simulink model "ebike_UB_2"  (Simulink 8.5)
settings: Solver=ode3  StartTime=0.0  StopTime=0.5  FixedStep=0.001  MaxStep=0.001  MinStep=0.001  RelTol=1e-3
values from neighbouring files (symbols this model uses):
  air_density = 1.225    [run_sim.m]
  air_drag_coeff = 0.4    [run_sim.m]
  frontal_area = 0.38    [run_sim.m]
  gravity = 9.8    [run_sim.m]
  rolling_fric_coeff = 0.003    [run_sim.m]
  vehicle_mass = driver_mass+bike_mass    (= 82)    [run_sim.m]
libraries: simulink x1
settings Model: Creator=stwei  LastModifiedBy=bolatu
settings DataIOCC: SignalLoggingSaveFormat=Dataset  SaveOutput=off  ReturnWorkspaceOutputs=on
settings DebuggingCC: SolverPrmCheckMsg=warning  FcnCallInpInsideContextMsg=UseLocalSettings

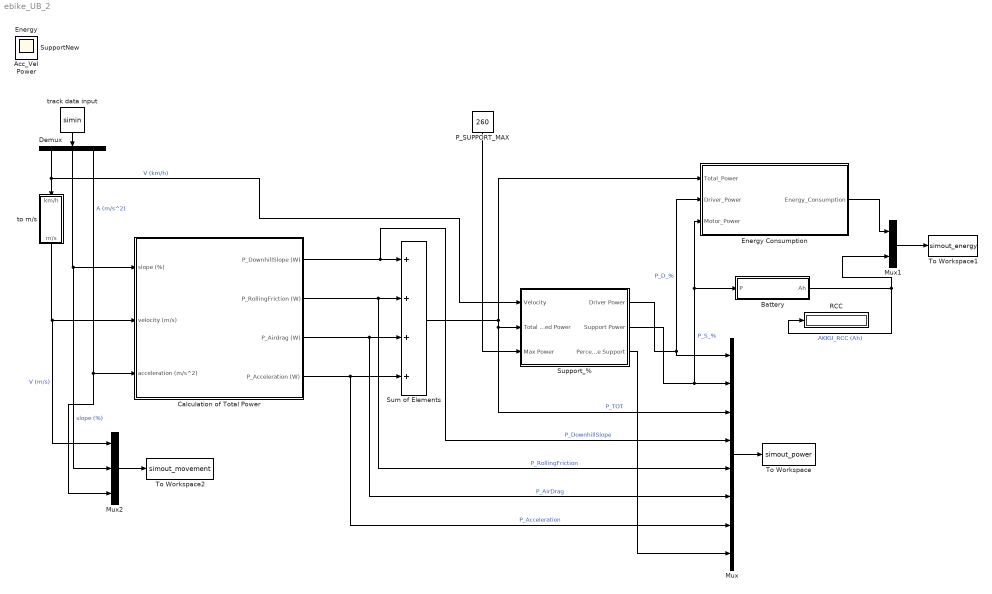
== system ebike_UB_2 ==
  Battery : Subsystem
  Calculation of Total Power : Subsystem
  Demux : Demux  Outputs=3
  Energy Consumption : Subsystem
  Mux : Mux  Inputs=8
  Mux1 : Mux  Inputs=2
  Mux2 : Mux  Inputs=3
  P_SUPPORT_MAX : Constant  Value=260
  RCC : Display
  Sum of Elements : Sum  Inputs=++++
  Support_% : Subsystem
  To Workspace : ToWorkspace  VariableName=simout_power  SaveFormat=Timeseries  SampleTime=-1
  To Workspace1 : ToWorkspace  VariableName=simout_energy  SaveFormat=Timeseries  SampleTime=-1
  To Workspace2 : ToWorkspace  VariableName=simout_movement  SaveFormat=Timeseries  SampleTime=-1
  to m/s : Subsystem
  track data input : FromWorkspace  VariableName=simin  SampleTime=0  OutputAfterFinalValue=Setting to zero
  Acc_Vel : Scope  NumInputPorts=4
      settings: ShowLegends=on  YMin=-5~-5~-5~-5  YMax=5~5~5~5
  Energy : Scope
      settings: ShowLegends=on  SaveName=ScopeData2
  Power : Scope
      settings: ShowLegends=on
  SupportNew : Scope  NumInputPorts=3
      settings: ShowLegends=on  YMin=-5~-5~-5  YMax=5~5~5  SaveName=ScopeData3
  wires:
  P_SUPPORT_MAX/1 -> Support_%/3(Max Power)
  track data input/1 -> Demux/1
  Demux/1 -> to m/s/1(km/h), Support_%/1(Velocity)  "V (km/h)"
  Demux/2 -> Mux2/2, Calculation of Total Power/1(slope (%))  "slope (%)"
  to m/s/1(m/s) -> Mux2/1, Calculation of Total Power/2(velocity (m/s))  "V (m/s)"
  Sum of Elements/1 -> Mux/3, Support_%/2(Total Needed Power), Energy Consumption/1(Total_Power)  "P_TOT"
  Calculation of Total Power/1(P_DownhillSlope (W)) -> Mux/4, Sum of Elements/1  "P_DownhillSlope"
  Calculation of Total Power/2(P_RollingFriction (W)) -> Mux/5, Sum of Elements/2  "P_RollingFriction"
  Calculation of Total Power/3(P_Airdrag (W)) -> Mux/6, Sum of Elements/3  "P_AirDrag"
  Calculation of Total Power/4(P_Acceleration (W)) -> Mux/7, Sum of Elements/4  "P_Acceleration"
  Demux/3 -> Mux2/3, Calculation of Total Power/3(acceleration (m/s^2))  "A (m/s^2)"
  Mux/1 -> To Workspace/1
  Support_%/2(Support Power) -> Energy Consumption/3(Motor_Power), Battery/1(P), Mux/2  "P_S_%"
  Support_%/1(Driver Power) -> Mux/1, Energy Consumption/2(Driver_Power)  "P_D_%"
  Energy Consumption/1(Energy_Consumption) -> Mux1/1
  Battery/1(Ah) -> RCC/1, Mux1/2  "AKKU_RCC (Ah)"
  Mux1/1 -> To Workspace1/1
  Mux2/1 -> To Workspace2/1
  Support_%/3(Percentage Support) -> Mux/8

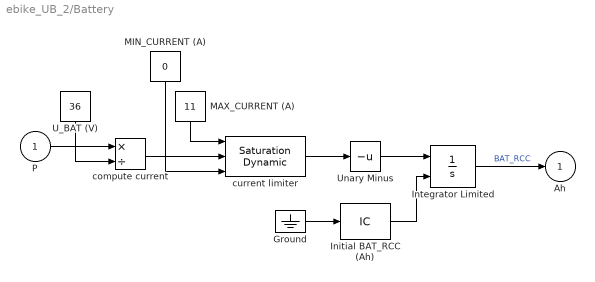
== system ebike_UB_2/Battery ==
  P : Inport
  Ground : Ground
  Initial BAT_RCC (Ah) : InitialCondition  Value=11
  Integrator Limited : Integrator  InitialConditionSource=external  LimitOutput=on  UpperSaturationLimit=13  LowerSaturationLimit=0
  MAX_CURRENT (A) : Constant  Value=11
  MIN_CURRENT (A) : Constant  Value=0
  U_BAT (V) : Constant  Value=36
  Unary Minus : UnaryMinus
  compute current : Product  Inputs=*/
  current limiter : simulink/Discontinuities/Saturation Dynamic  OutMin=[]  OutMax=[]  OutDataTypeStr=Inherit: Same as second input  OutDataType=fixdt(1, 16)  OutScaling=2^-10  DoSatur=on
  Ah : Outport
  wires:
  Ground/1 -> Initial BAT_RCC (Ah)/1
  U_BAT (V)/1 -> compute current/2
  Initial BAT_RCC (Ah)/1 -> Integrator Limited/2
  Unary Minus/1 -> Integrator Limited/1
  P/1 -> compute current/1
  Integrator Limited/1 -> Ah/1  "BAT_RCC"
  current limiter/1 -> Unary Minus/1
  compute current/1 -> current limiter/2
  MAX_CURRENT (A)/1 -> current limiter/1
  MIN_CURRENT (A)/1 -> current limiter/3

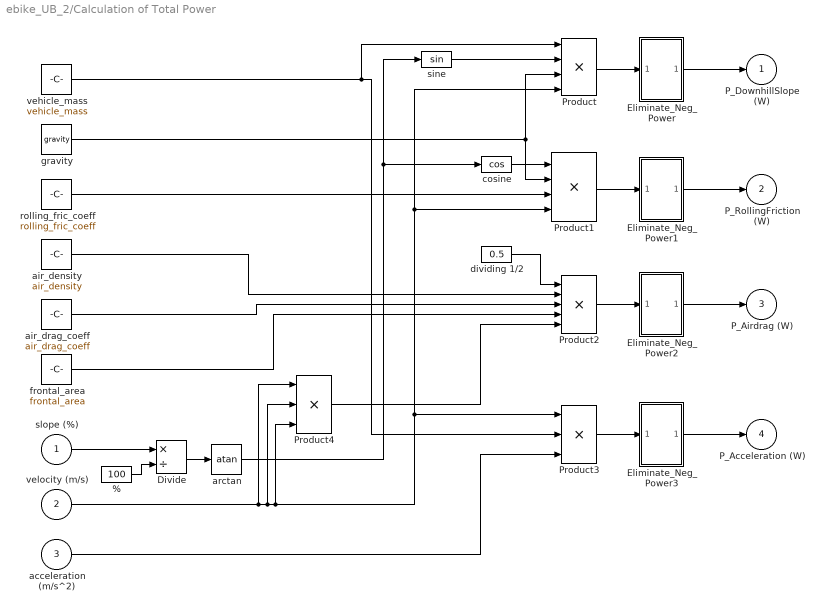
== system ebike_UB_2/Calculation of Total Power ==
  slope (%) : Inport
  velocity (m/s) : Inport  Port=2
  acceleration (m/s^2) : Inport  Port=3
  % : Constant  Value=100
  Divide : Product  Inputs=*/
  Eliminate_Neg_Power : Subsystem
  Eliminate_Neg_Power1 : Subsystem
  Eliminate_Neg_Power2 : Subsystem
  Eliminate_Neg_Power3 : Subsystem
  Product : Product  Inputs=4
  Product1 : Product  Inputs=4
  Product2 : Product  Inputs=5
  Product3 : Product  Inputs=3
  Product4 : Product  Inputs=3
  air_density : Constant  Value=air_density
  air_drag_coeff : Constant  Value=air_drag_coeff
  arctan : Trigonometry  Operator=atan
  cosine : Trigonometry  Operator=cos
  dividing 1/2 : Constant  Value=0.5
  frontal_area : Constant  Value=frontal_area
  gravity : Constant  Value=gravity
  rolling_fric_coeff : Constant  Value=rolling_fric_coeff
  sine : Trigonometry
  vehicle_mass : Constant  Value=vehicle_mass
  P_DownhillSlope (W) : Outport
  P_RollingFriction (W) : Outport  Port=2
  P_Airdrag (W) : Outport  Port=3
  P_Acceleration (W) : Outport  Port=4
  wires:
  slope (%)/1 -> Divide/1
  %/1 -> Divide/2
  Divide/1 -> arctan/1
  vehicle_mass/1 -> Product/1, Product3/2
  gravity/1 -> Product/3, Product1/2
  sine/1 -> Product/2
  arctan/1 -> sine/1, cosine/1
  velocity (m/s)/1 -> Product3/1, Product/4, Product1/4, Product4/3, Product4/2, Product4/1
  Product1/1 -> Eliminate_Neg_Power1/1(In1)
  cosine/1 -> Product1/1
  rolling_fric_coeff/1 -> Product1/3
  acceleration (m/s^2)/1 -> Product3/3
  air_density/1 -> Product2/2
  air_drag_coeff/1 -> Product2/3
  frontal_area/1 -> Product2/4
  Product4/1 -> Product2/5
  dividing 1/2/1 -> Product2/1
  Product/1 -> Eliminate_Neg_Power/1(In1)
  Eliminate_Neg_Power/1(Out1) -> P_DownhillSlope (W)/1
  Eliminate_Neg_Power1/1(Out1) -> P_RollingFriction (W)/1
  Product2/1 -> Eliminate_Neg_Power2/1(In1)
  Eliminate_Neg_Power2/1(Out1) -> P_Airdrag (W)/1
  Product3/1 -> Eliminate_Neg_Power3/1(In1)
  Eliminate_Neg_Power3/1(Out1) -> P_Acceleration (W)/1

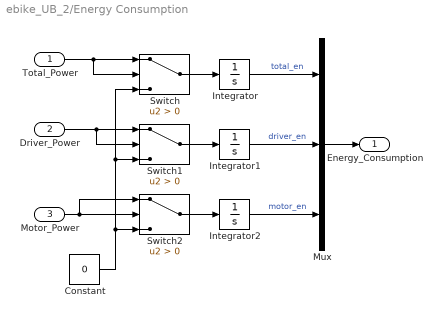
== system ebike_UB_2/Energy Consumption ==
  Total_Power : Inport
  Driver_Power : Inport  Port=2
  Motor_Power : Inport  Port=3
  Constant : Constant  Value=0
  Integrator : Integrator
  Integrator1 : Integrator
  Integrator2 : Integrator
  Mux : Mux  Inputs=3
  Switch : Switch  Criteria=u2 > Threshold
  Switch1 : Switch  Criteria=u2 > Threshold
  Switch2 : Switch  Criteria=u2 > Threshold
  Energy_Consumption : Outport
  wires:
  Switch2/1 -> Integrator2/1
  Switch1/1 -> Integrator1/1
  Switch/1 -> Integrator/1
  Integrator/1 -> Mux/1  "total_en"
  Integrator1/1 -> Mux/2  "driver_en"
  Integrator2/1 -> Mux/3  "motor_en"
  Mux/1 -> Energy_Consumption/1
  Total_Power/1 -> Switch/2, Switch/1
  Driver_Power/1 -> Switch1/2, Switch1/1
  Motor_Power/1 -> Switch2/1, Switch2/2
  Constant/1 -> Switch/3, Switch1/3, Switch2/3

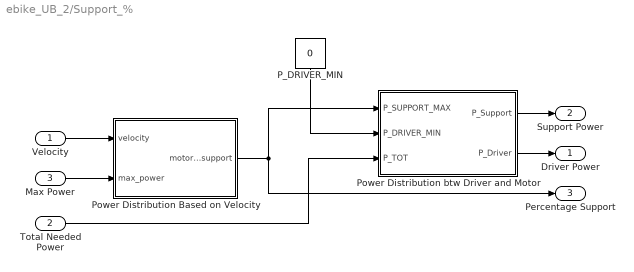
== system ebike_UB_2/Support_% ==
  Velocity : Inport
  Total Needed Power : Inport  Port=2
  Max Power : Inport  Port=3
  P_DRIVER_MIN : Constant  Value=0
  Power Distribution Based on Velocity : Subsystem
  Power Distribution btw Driver and Motor : Subsystem
  Driver Power : Outport
  Support Power : Outport  Port=2
  Percentage Support : Outport  Port=3
  wires:
  Total Needed Power/1 -> Power Distribution btw Driver and Motor/3(P_TOT)
  P_DRIVER_MIN/1 -> Power Distribution btw Driver and Motor/2(P_DRIVER_MIN)
  Power Distribution Based on Velocity/1(motor_support) -> Power Distribution btw Driver and Motor/1(P_SUPPORT_MAX), Percentage Support/1
  Power Distribution btw Driver and Motor/1(P_Support) -> Support Power/1
  Power Distribution btw Driver and Motor/2(P_Driver) -> Driver Power/1
  Max Power/1 -> Power Distribution Based on Velocity/2(max_power)
  Velocity/1 -> Power Distribution Based on Velocity/1(velocity)

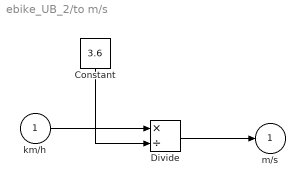
== system ebike_UB_2/to m/s ==
  km/h : Inport
  Constant : Constant  Value=3.6
  Divide : Product  Inputs=*/
  m/s : Outport
  wires:
  Constant/1 -> Divide/2
  km/h/1 -> Divide/1
  Divide/1 -> m/s/1

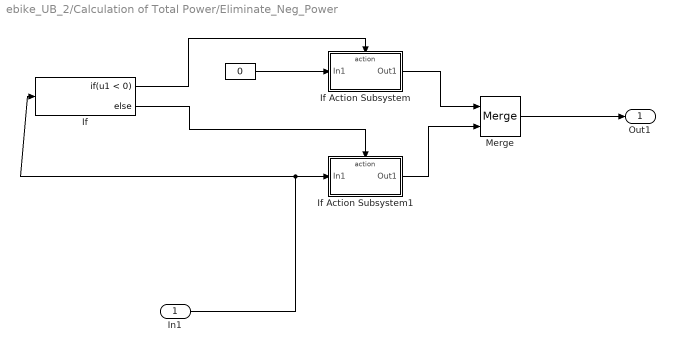
== system ebike_UB_2/Calculation of Total Power/Eliminate_Neg_Power ==
  In1 : Inport
  " " : Constant  Value=0
  If : If  IfExpression=u1 < 0
  If Action Subsystem : Subsystem  TreatAsAtomicUnit=on
  If Action Subsystem1 : Subsystem  TreatAsAtomicUnit=on
  Merge : Merge
  Out1 : Outport
  wires:
  If Action Subsystem1/1(Out1) -> Merge/2
  If/2 -> If Action Subsystem1/Action
  If Action Subsystem/1(Out1) -> Merge/1
  Merge/1 -> Out1/1
  " "/1 -> If Action Subsystem/1(In1)
  In1/1 -> If Action Subsystem1/1(In1), If/1
  If/1 -> If Action Subsystem/Action

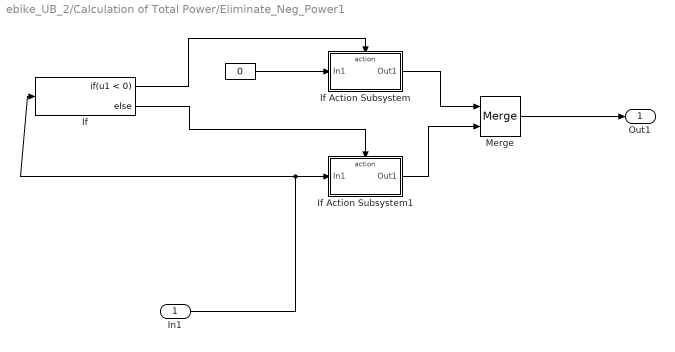
== system ebike_UB_2/Calculation of Total Power/Eliminate_Neg_Power1 ==
  In1 : Inport
  " " : Constant  Value=0
  If : If  IfExpression=u1 < 0
  If Action Subsystem : Subsystem  TreatAsAtomicUnit=on
  If Action Subsystem1 : Subsystem  TreatAsAtomicUnit=on
  Merge : Merge
  Out1 : Outport
  wires:
  If Action Subsystem1/1(Out1) -> Merge/2
  If/2 -> If Action Subsystem1/Action
  If Action Subsystem/1(Out1) -> Merge/1
  Merge/1 -> Out1/1
  " "/1 -> If Action Subsystem/1(In1)
  In1/1 -> If Action Subsystem1/1(In1), If/1
  If/1 -> If Action Subsystem/Action

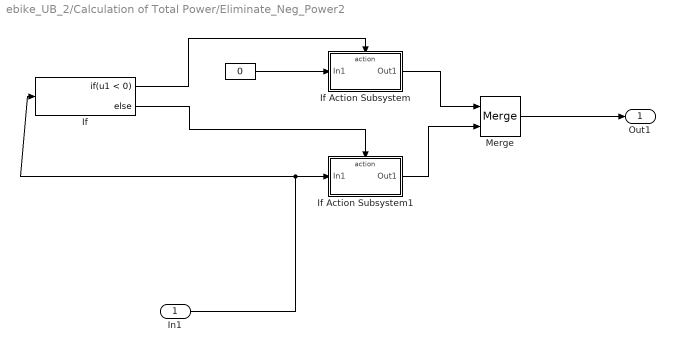
== system ebike_UB_2/Calculation of Total Power/Eliminate_Neg_Power2 ==
  In1 : Inport
  " " : Constant  Value=0
  If : If  IfExpression=u1 < 0
  If Action Subsystem : Subsystem  TreatAsAtomicUnit=on
  If Action Subsystem1 : Subsystem  TreatAsAtomicUnit=on
  Merge : Merge
  Out1 : Outport
  wires:
  If Action Subsystem1/1(Out1) -> Merge/2
  If/2 -> If Action Subsystem1/Action
  If Action Subsystem/1(Out1) -> Merge/1
  Merge/1 -> Out1/1
  " "/1 -> If Action Subsystem/1(In1)
  In1/1 -> If Action Subsystem1/1(In1), If/1
  If/1 -> If Action Subsystem/Action

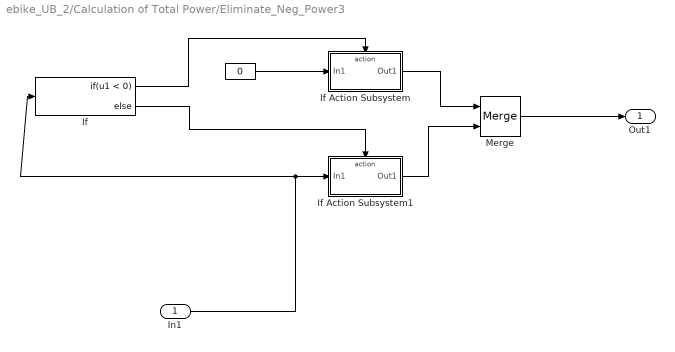
== system ebike_UB_2/Calculation of Total Power/Eliminate_Neg_Power3 ==
  In1 : Inport
  " " : Constant  Value=0
  If : If  IfExpression=u1 < 0
  If Action Subsystem : Subsystem  TreatAsAtomicUnit=on
  If Action Subsystem1 : Subsystem  TreatAsAtomicUnit=on
  Merge : Merge
  Out1 : Outport
  wires:
  If Action Subsystem1/1(Out1) -> Merge/2
  If/2 -> If Action Subsystem1/Action
  If Action Subsystem/1(Out1) -> Merge/1
  Merge/1 -> Out1/1
  " "/1 -> If Action Subsystem/1(In1)
  In1/1 -> If Action Subsystem1/1(In1), If/1
  If/1 -> If Action Subsystem/Action

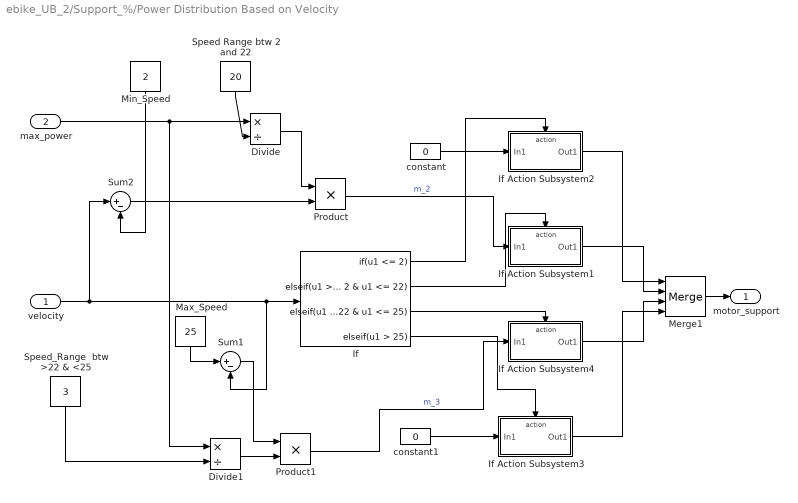
== system ebike_UB_2/Support_%/Power Distribution Based on Velocity ==
  velocity : Inport
  max_power : Inport  Port=2
  " constant" : Constant  Value=0
  " constant1" : Constant  Value=0
  Divide : Product  Inputs=*/
  Divide1 : Product  Inputs=*/
  If : If  IfExpression=u1 <= 2  ElseIfExpressions=u1 > 2 & u1 <= 22, u1 > 22 & u1 <= 25, u1 > 25  ShowElse=off
  If Action Subsystem1 : Subsystem  TreatAsAtomicUnit=on
  If Action Subsystem2 : Subsystem  TreatAsAtomicUnit=on
  If Action Subsystem3 : Subsystem  TreatAsAtomicUnit=on
  If Action Subsystem4 : Subsystem  TreatAsAtomicUnit=on
  Max_Speed : Constant  Value=25
  Merge1 : Merge  Inputs=4
  Min_Speed : Constant  Value=2
  Product : Product
  Product1 : Product
  Speed Range btw 2 and 22 : Constant  Value=20
  Speed_Range  btw >22 & <25 : Constant  Value=3
  Sum1 : Sum  Inputs=|+-
  Sum2 : Sum  Inputs=|+-
  motor_support : Outport
  wires:
  velocity/1 -> Sum2/1, If/1, Sum1/2
  " constant"/1 -> If Action Subsystem2/1(In1)
  If/1 -> If Action Subsystem2/Action
  " constant1"/1 -> If Action Subsystem3/1(In1)
  Speed Range btw 2 and 22/1 -> Divide/2
  Divide/1 -> Product/1
  If/2 -> If Action Subsystem1/Action
  If/3 -> If Action Subsystem4/Action
  If/4 -> If Action Subsystem3/Action
  If Action Subsystem2/1(Out1) -> Merge1/1
  If Action Subsystem3/1(Out1) -> Merge1/4
  max_power/1 -> Divide/1, Divide1/1
  Max_Speed/1 -> Sum1/1
  Speed_Range  btw >22 & <25/1 -> Divide1/2
  Divide1/1 -> Product1/2
  Sum1/1 -> Product1/1
  Merge1/1 -> motor_support/1
  Product/1 -> If Action Subsystem1/1(In1)  "m_2"
  Product1/1 -> If Action Subsystem4/1(In1)  "m_3"
  If Action Subsystem4/1(Out1) -> Merge1/3
  If Action Subsystem1/1(Out1) -> Merge1/2
  Min_Speed/1 -> Sum2/2
  Sum2/1 -> Product/2

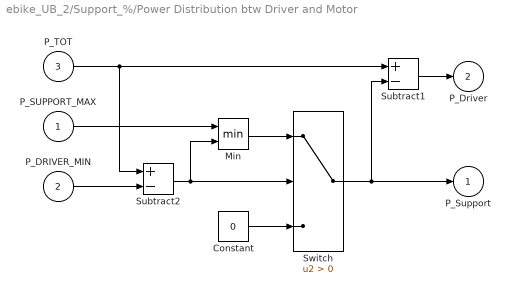
== system ebike_UB_2/Support_%/Power Distribution btw Driver and Motor ==
  P_SUPPORT_MAX : Inport
  P_DRIVER_MIN : Inport  Port=2
  P_TOT : Inport  Port=3
  Constant : Constant  Value=0
  Min : MinMax  Inputs=2
  Subtract1 : Sum  Inputs=+-
  Subtract2 : Sum  Inputs=+-
  Switch : Switch  Criteria=u2 > Threshold
  P_Support : Outport
  P_Driver : Outport  Port=2
  wires:
  P_TOT/1 -> Subtract1/1, Subtract2/1
  Subtract1/1 -> P_Driver/1
  Subtract2/1 -> Switch/2, Min/2
  P_SUPPORT_MAX/1 -> Min/1
  P_DRIVER_MIN/1 -> Subtract2/2
  Min/1 -> Switch/1
  Switch/1 -> P_Support/1, Subtract1/2
  Constant/1 -> Switch/3

== system ebike_UB_2/Calculation of Total Power/Eliminate_Neg_Power/If Action Subsystem ==
  In1 : Inport
  Action Port : ActionPort  ActionType=then
  Out1 : Outport
  wires:
  In1/1 -> Out1/1

== system ebike_UB_2/Calculation of Total Power/Eliminate_Neg_Power/If Action Subsystem1 ==
  In1 : Inport
  Action Port : ActionPort  ActionType=else
  Out1 : Outport
  wires:
  In1/1 -> Out1/1

== system ebike_UB_2/Calculation of Total Power/Eliminate_Neg_Power1/If Action Subsystem ==
  In1 : Inport
  Action Port : ActionPort  ActionType=then
  Out1 : Outport
  wires:
  In1/1 -> Out1/1

== system ebike_UB_2/Calculation of Total Power/Eliminate_Neg_Power1/If Action Subsystem1 ==
  In1 : Inport
  Action Port : ActionPort  ActionType=else
  Out1 : Outport
  wires:
  In1/1 -> Out1/1

== system ebike_UB_2/Calculation of Total Power/Eliminate_Neg_Power2/If Action Subsystem ==
  In1 : Inport
  Action Port : ActionPort  ActionType=then
  Out1 : Outport
  wires:
  In1/1 -> Out1/1

== system ebike_UB_2/Calculation of Total Power/Eliminate_Neg_Power2/If Action Subsystem1 ==
  In1 : Inport
  Action Port : ActionPort  ActionType=else
  Out1 : Outport
  wires:
  In1/1 -> Out1/1

== system ebike_UB_2/Calculation of Total Power/Eliminate_Neg_Power3/If Action Subsystem ==
  In1 : Inport
  Action Port : ActionPort  ActionType=then
  Out1 : Outport
  wires:
  In1/1 -> Out1/1

== system ebike_UB_2/Calculation of Total Power/Eliminate_Neg_Power3/If Action Subsystem1 ==
  In1 : Inport
  Action Port : ActionPort  ActionType=else
  Out1 : Outport
  wires:
  In1/1 -> Out1/1

== system ebike_UB_2/Support_%/Power Distribution Based on Velocity/If Action Subsystem1 ==
  In1 : Inport
  Action Port : ActionPort  ActionType=elseif
  Out1 : Outport
  wires:
  In1/1 -> Out1/1

== system ebike_UB_2/Support_%/Power Distribution Based on Velocity/If Action Subsystem2 ==
  In1 : Inport
  Action Port : ActionPort  ActionType=then
  Out1 : Outport
  wires:
  In1/1 -> Out1/1

== system ebike_UB_2/Support_%/Power Distribution Based on Velocity/If Action Subsystem3 ==
  In1 : Inport
  Action Port : ActionPort  ActionType=elseif
  Out1 : Outport
  wires:
  In1/1 -> Out1/1

== system ebike_UB_2/Support_%/Power Distribution Based on Velocity/If Action Subsystem4 ==
  In1 : Inport
  Action Port : ActionPort  ActionType=elseif
  Out1 : Outport
  wires:
  In1/1 -> Out1/1
